simulink model "sim"  (R2024b)
settings: Solver=VariableStepAuto  StartTime=0.0  StopTime=10.0  RelTol=1e-3
libraries: slpidlib x1
settings Model: Creator=nhola  LastModifiedBy=nhola

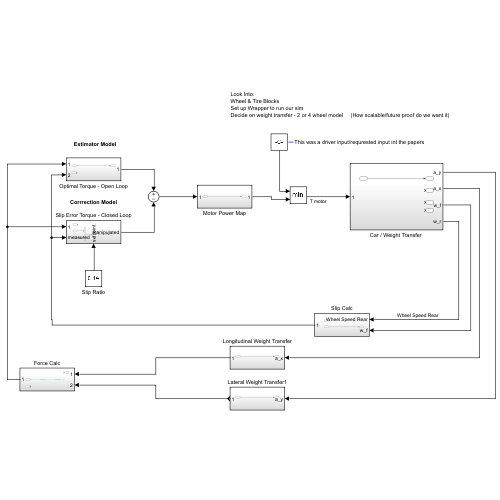
[thumbnail: Simulink's stored preview of the top-level diagram]
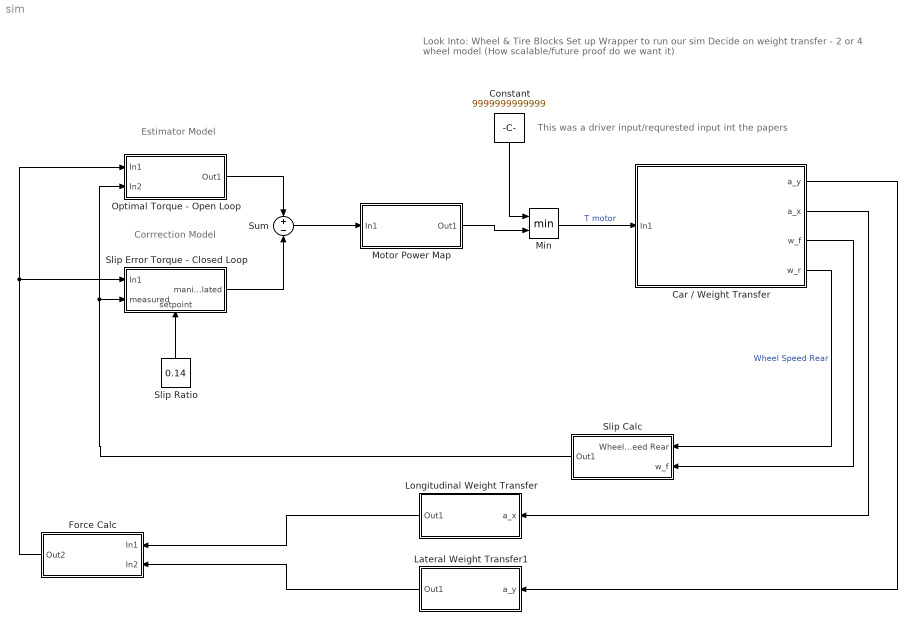
== system sim ==
  note: This was a driver input/requrested input int the papers
  note: Estimator Model
  note: Corrrection Model
  note: Look Into:
      | Wheel & Tire Blocks
      | Set up Wrapper to run our sim
      | Decide on weight transfer - 2 or 4 wheel model	(How scalable/future proof do we want it)
  "Car / Weight Transfer " : Subsystem
  Constant : Constant  Value=9999999999999
  Force Calc : Subsystem
  Lateral Weight Transfer1 : Subsystem
  Longitudinal Weight Transfer : Subsystem
  Min : MinMax  Inputs=2
  Motor Power Map : Subsystem
  Optimal Torque - Open Loop : Subsystem
  Slip Calc : Subsystem
  Slip Error Torque - Closed Loop : Subsystem
      settings: PortSchema="{\"entries\":[{\"content\":{\"sides\":[{\"content\":{\"connectorIds\":[\"In1\",\"In2\"]},\"type\":\"ConnectorPlacement.EquallySpacedRectSide\",\"uuid\":\"2e14bde7-f8d2-4eed-92ee-ce4e5654d4f8\"},{\"content\":{\"connectorIds\":[\"Out1\"],\"side\":\"RIGHT\"},\"type\":\"ConnectorPlacement.EquallySpacedRectSide\",\"uuid\":\"a3be9eae-ada7-4228-af9a-31d1d8dc2318\"},{\"content\":{\"side\":\"TOP\"},\"type\":\"ConnectorPlacement.EquallySpacedRectSide\",\"uuid\":\"1940a9a7-18ed-4824-a95e-5036d1b3bdfe\"},{\"content\":{\"connectorIds\":[\"In3\"],\"side\":\"BOTTOM\"},\"type\":\"ConnectorPlacement.EquallySpacedRectSide\",\"uuid\":\"003842a2-1238-44c6-9c91-e165d329f765\"}]},\"type\":\"ConnectorPlacement.EquallySpacedConnector\",\"uuid\":\"2a624467-2fbe-40cb-bd4c-f92ddee7aaab\"}],\"packageUris\":[\"http://schema.mathworks.com/mf0/Connector/R2020b\"],\"version\":\"1.0\"}"
  Slip Ratio : Constant  Value=0.14
  Sum : Sum  Inputs=+-
  wires:
  Min/1 -> "Car / Weight Transfer "/1(In1)  "T motor"
  "Car / Weight Transfer "/2(a_x) -> Longitudinal Weight Transfer/1(a_x)
  "Car / Weight Transfer "/4(w_r) -> Slip Calc/1(Wheel Speed Rear)  "Wheel Speed Rear"
  "Car / Weight Transfer "/1(a_y) -> Lateral Weight Transfer1/1(a_y)
  "Car / Weight Transfer "/3(w_f) -> Slip Calc/2(w_f)
  Longitudinal Weight Transfer/1(Out1) -> Force Calc/1(In1)
  Lateral Weight Transfer1/1(Out1) -> Force Calc/2(In2)
  Slip Ratio/1 -> Slip Error Torque - Closed Loop/3(setpoint)
  Slip Calc/1(Out1) -> Optimal Torque - Open Loop/2(In2), Slip Error Torque - Closed Loop/2(measured)
  Force Calc/1(Out2) -> Optimal Torque - Open Loop/1(In1), Slip Error Torque - Closed Loop/1(In1)
  Optimal Torque - Open Loop/1(Out1) -> Sum/1
  Slip Error Torque - Closed Loop/1(manipulated) -> Sum/2
  Motor Power Map/1(Out1) -> Min/2
  Sum/1 -> Motor Power Map/1(In1)
  Constant/1 -> Min/1

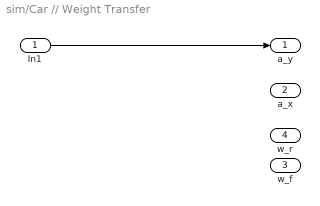
== system sim/Car // Weight Transfer  ==
  In1 : Inport
  a_y : Outport
  a_x : Outport  Port=2
  w_f : Outport  Port=3
  w_r : Outport  Port=4
  wires:
  In1/1 -> a_y/1

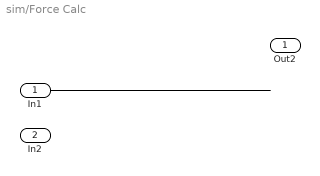
== system sim/Force Calc ==
  In1 : Inport
  In2 : Inport  Port=2
  Out2 : Outport
  wires:
  In1/1 -> ?

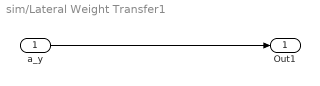
== system sim/Lateral Weight Transfer1 ==
  a_y : Inport
  Out1 : Outport
  wires:
  a_y/1 -> Out1/1

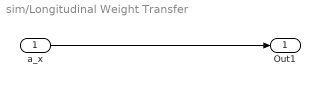
== system sim/Longitudinal Weight Transfer ==
  a_x : Inport
  Out1 : Outport
  wires:
  a_x/1 -> Out1/1

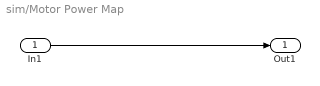
== system sim/Motor Power Map ==
  In1 : Inport
  Out1 : Outport
  wires:
  In1/1 -> Out1/1

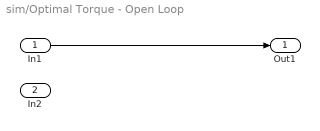
== system sim/Optimal Torque - Open Loop ==
  In1 : Inport
  In2 : Inport  Port=2
  Out1 : Outport
  wires:
  In1/1 -> Out1/1

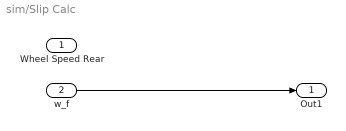
== system sim/Slip Calc ==
  Wheel Speed Rear : Inport
  w_f : Inport  Port=2
  Out1 : Outport
  wires:
  w_f/1 -> Out1/1

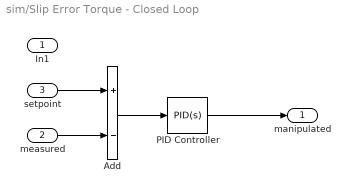
== system sim/Slip Error Torque - Closed Loop ==
  In1 : Inport
  measured : Inport  Port=2
  setpoint : Inport  Port=3
  Add : Sum  Inputs=+-
  PID Controller : slpidlib/PID Controller  Controller=PID  Form=Parallel  TimeDomain=Continuous-time  UseExternalTs=off  SampleTime=-1  IntegratorMethod=Forward Euler  FilterMethod=Forward Euler  ControllerParametersSource=internal  P=1  I=1  UseKiTs=off  D=0  UseExternalDerivativeSource=off  N=100  UseFilter=on  TunerSelectOption=Transfer Function Based (PID Tuner App)  InitialConditionSource=internal  InitialConditionForIntegrator=0  InitialConditionForFilter=0  DifferentiatorICPrevScaledInput=0  ExternalReset=none  TrackingMode=off  Kt=1  LimitOutput=off  SatLimitsSource=internal  UpperSaturationLimit=inf  LowerSaturationLimit=-inf  LinearizeAsGain=on  AntiWindupMode=none  Kb=1  LimitIntegrator=off  UpperIntegratorSaturationLimit=inf  LowerIntegratorSaturationLimit=-inf  POutMin=[]  POutMax=[]  IOutMin=[]  IOutMax=[]  DOutMin=[]  DOutMax=[]  NOutMin=[]  NOutMax=[]  SumOutMin=[]  SumOutMax=[]  SaturationOutMin=[]  SaturationOutMax=[]  PParamMin=[]  PParamMax=[]  IParamMin=[]  IParamMax=[]  DParamMin=[]  DParamMax=[]  NParamMin=[]  NParamMax=[]  KbParamMin=[]  KbParamMax=[]  KtParamMin=[]  KtParamMax=[]  KbOutMin=[]  KbOutMax=[]  KtOutMin=[]  KtOutMax=[]  IntegratorOutMin=[]  IntegratorOutMax=[]  FilterOutMin=[]  FilterOutMax=[]  SumI1OutMin=[]  SumI1OutMax=[]  SumI2OutMin=[]  SumI2OutMax=[]  SumI3OutMin=[]  SumI3OutMax=[]  SumI4OutMin=[]  SumI4OutMax=[]  SumDOutMin=[]  SumDOutMax=[]  DifferentiatorOutMin=[]  DifferentiatorOutMax=[]  FilterDiffOutCoefMin=[]  FilterDiffOutCoefMax=[]  ReciprocalOutMin=[]  ReciprocalOutMax=[]  SumDenOutMin=[]  SumDenOutMax=[]  SumNumOutMin=[]  SumNumOutMax=[]  DivideOutMin=[]  DivideOutMax=[]  UdiffTsProdOutMin=[]  UdiffTsProdOutMax=[]  NTsProdOutMin=[]  NTsProdOutMax=[]  UintegralTsProdOutMin=[]  UintegralTsProdOutMax=[]  UngainTsProdOutMin=[]  UngainTsProdOutMax=[]  ClampingZeroOutDataTypeStr=Inherit: Inherit via back propagation  ClampingZeroOutMin=[]  ClampingZeroOutMax=[]  FilterDenConstantOutDataTypeStr=Inherit: Inherit via back propagation  FilterDenConstantOutMin=[]  FilterDenConstantOutMax=[]  PCopyOutDataTypeStr=Inherit: Inherit via back propagation  PCopyOutMin=[]  PCopyOutMax=[]  NCopyOutDataTypeStr=Inherit: Inherit via back propagation  NCopyOutMin=[]  NCopyOutMax=[]  IntegratorContinuousStateAttributes=''  IntegratorStateMustResolveToSignalObject=off  IntegratorRTWStateStorageClass=Auto  FilterContinuousStateAttributes=''  FilterStateMustResolveToSignalObject=off  FilterRTWStateStorageClass=Auto  ParallelPVariant=InternalParameters  IdealPVariant=Disabled  IVariant=InternalParameters  DVariant=InternalParameters  IntegratorVariant=Continuous  SatVariant=Disabled  AWVariant=Passthrough  PCopyVariant=Disabled  TRVariant=Disabled  FdbkBlocksVariant=Forward  IdealPFdbkVariant=Disabled  SatFdbkVariant=Disabled  DerivativeFilterVariant=ContFilter  NVariant=InternalParameters  NCopyVariant=Disabled  FilterICVariant=InternalICsFilter  IntegratorICVariant=InternalICs  ExternalResetVariant=Disabled  TRSumVariant=Passthrough  SumFdbkVariant=Disabled  SumVariant=Sum_PID  TsampFilterVariant=InternalTs  TsampNgainVariant=Passthrough  TsampIntegralVariant=Disabled_SignalSpec  ExternalSaturationOutDataTypeStr=Inherit: Same as second input  DerivativeSourceVariant=ErrorSignal  PreIntVariant=InternalPreInt
  manipulated : Outport
  wires:
  setpoint/1 -> Add/1
  measured/1 -> Add/2
  Add/1 -> PID Controller/1
  PID Controller/1 -> manipulated/1
